simulink model "pid_simulink"  (R2014b)
settings: Solver=ode45  StartTime=0.0  StopTime=10  RelTol=1e-3
values from neighbouring files (symbols this model uses):
  Bm = 0.01    [d_1_dc_motor_parameter.m]    (also in d_2_draw_wt_theta_real.m; d_2_draw_wt_theta_tf.m; d_4_dc_motor_bar_parameter.m; plot.m)
  Jm = 0.000052    (= 5.2e-05)    [d_1_dc_motor_parameter.m]    (also in d_2_draw_wt_theta_real.m; d_2_draw_wt_theta_tf.m; d_4_dc_motor_bar_parameter.m; plot.m)
  Ke = 0.235    [d_1_dc_motor_parameter.m]    (also in d_2_draw_wt_theta_real.m; d_2_draw_wt_theta_tf.m; d_4_dc_motor_bar_parameter.m; plot.m)
  Kt = 0.235    [d_1_dc_motor_parameter.m]    (also in d_2_draw_wt_theta_real.m; d_2_draw_wt_theta_tf.m; d_4_dc_motor_bar_parameter.m; plot.m)
  La = 0.23    [d_1_dc_motor_parameter.m]    (also in d_2_draw_wt_theta_real.m; d_2_draw_wt_theta_tf.m; d_4_dc_motor_bar_parameter.m; plot.m)
  Ra = 2    [d_1_dc_motor_parameter.m]    (also in d_2_draw_wt_theta_real.m; d_2_draw_wt_theta_tf.m; d_4_dc_motor_bar_parameter.m; plot.m)
libraries: simulink x3
settings Model: Creator=Admin  LastModifiedBy=Admin

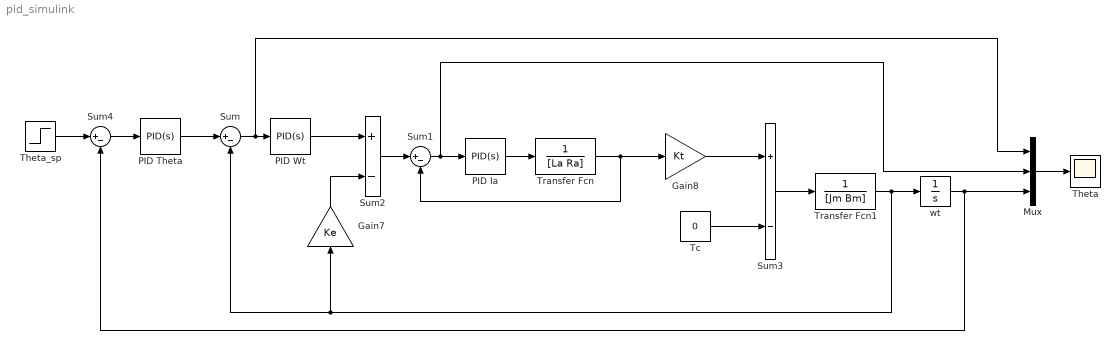
== system pid_simulink ==
  Gain7 : Gain  Gain=Ke
  Gain8 : Gain  Gain=Kt
  Mux : Mux  Inputs=3
  PID Ia : simulink/Continuous/PID Controller  Controller=PID  TimeDomain=Continuous-time  SampleTime=-1  IntegratorMethod=Forward Euler  FilterMethod=Forward Euler  Form=Parallel  P=0.2  I=0.4  D=0  N=0  InitialConditionSource=internal  InitialConditionForIntegrator=0  InitialConditionForFilter=0  ExternalReset=none  LimitOutput=off  UpperSaturationLimit=inf  LowerSaturationLimit=-inf  LinearizeAsGain=on  AntiWindupMode=none  Kb=1  TrackingMode=off  Kt=1  PParamMin=[]  PParamMax=[]  IParamMin=[]  IParamMax=[]  DParamMin=[]  DParamMax=[]  NParamMin=[]  NParamMax=[]  KbParamMin=[]  KbParamMax=[]  KtParamMin=[]  KtParamMax=[]  POutMin=[]  POutMax=[]  IOutMin=[]  IOutMax=[]  DOutMin=[]  DOutMax=[]  NOutMin=[]  NOutMax=[]  KbOutMin=[]  KbOutMax=[]  KtOutMin=[]  KtOutMax=[]  IntegratorOutMin=[]  IntegratorOutMax=[]  FilterOutMin=[]  FilterOutMax=[]  SumOutMin=[]  SumOutMax=[]  SumI1OutMin=[]  SumI1OutMax=[]  SumI2OutMin=[]  SumI2OutMax=[]  SumI3OutMin=[]  SumI3OutMax=[]  SumDOutMin=[]  SumDOutMax=[]  SaturationOutMin=[]  SaturationOutMax=[]  IntegratorContinuousStateAttributes=''  IntegratorStateMustResolveToSignalObject=off  IntegratorRTWStateStorageClass=Auto  FilterContinuousStateAttributes=''  FilterStateMustResolveToSignalObject=off  FilterRTWStateStorageClass=Auto  DifferentiatorICPrevScaledInput=0  DifferentiatorOutMin=[]  DifferentiatorOutMax=[]  UseFilter=on
  PID Theta : simulink/Continuous/PID Controller  Controller=PID  TimeDomain=Continuous-time  SampleTime=-1  IntegratorMethod=Forward Euler  FilterMethod=Forward Euler  Form=Parallel  P=10  I=0  D=0  N=0  InitialConditionSource=internal  InitialConditionForIntegrator=0  InitialConditionForFilter=0  ExternalReset=none  LimitOutput=off  UpperSaturationLimit=inf  LowerSaturationLimit=-inf  LinearizeAsGain=on  AntiWindupMode=none  Kb=1  TrackingMode=off  Kt=1  PParamMin=[]  PParamMax=[]  IParamMin=[]  IParamMax=[]  DParamMin=[]  DParamMax=[]  NParamMin=[]  NParamMax=[]  KbParamMin=[]  KbParamMax=[]  KtParamMin=[]  KtParamMax=[]  POutMin=[]  POutMax=[]  IOutMin=[]  IOutMax=[]  DOutMin=[]  DOutMax=[]  NOutMin=[]  NOutMax=[]  KbOutMin=[]  KbOutMax=[]  KtOutMin=[]  KtOutMax=[]  IntegratorOutMin=[]  IntegratorOutMax=[]  FilterOutMin=[]  FilterOutMax=[]  SumOutMin=[]  SumOutMax=[]  SumI1OutMin=[]  SumI1OutMax=[]  SumI2OutMin=[]  SumI2OutMax=[]  SumI3OutMin=[]  SumI3OutMax=[]  SumDOutMin=[]  SumDOutMax=[]  SaturationOutMin=[]  SaturationOutMax=[]  IntegratorContinuousStateAttributes=''  IntegratorStateMustResolveToSignalObject=off  IntegratorRTWStateStorageClass=Auto  FilterContinuousStateAttributes=''  FilterStateMustResolveToSignalObject=off  FilterRTWStateStorageClass=Auto  DifferentiatorICPrevScaledInput=0  DifferentiatorOutMin=[]  DifferentiatorOutMax=[]  UseFilter=on
  PID Wt : simulink/Continuous/PID Controller  Controller=PID  TimeDomain=Continuous-time  SampleTime=-1  IntegratorMethod=Forward Euler  FilterMethod=Forward Euler  Form=Parallel  P=1  I=2  D=0  N=0  InitialConditionSource=internal  InitialConditionForIntegrator=0  InitialConditionForFilter=0  ExternalReset=none  LimitOutput=off  UpperSaturationLimit=inf  LowerSaturationLimit=-inf  LinearizeAsGain=on  AntiWindupMode=none  Kb=1  TrackingMode=off  Kt=1  PParamMin=[]  PParamMax=[]  IParamMin=[]  IParamMax=[]  DParamMin=[]  DParamMax=[]  NParamMin=[]  NParamMax=[]  KbParamMin=[]  KbParamMax=[]  KtParamMin=[]  KtParamMax=[]  POutMin=[]  POutMax=[]  IOutMin=[]  IOutMax=[]  DOutMin=[]  DOutMax=[]  NOutMin=[]  NOutMax=[]  KbOutMin=[]  KbOutMax=[]  KtOutMin=[]  KtOutMax=[]  IntegratorOutMin=[]  IntegratorOutMax=[]  FilterOutMin=[]  FilterOutMax=[]  SumOutMin=[]  SumOutMax=[]  SumI1OutMin=[]  SumI1OutMax=[]  SumI2OutMin=[]  SumI2OutMax=[]  SumI3OutMin=[]  SumI3OutMax=[]  SumDOutMin=[]  SumDOutMax=[]  SaturationOutMin=[]  SaturationOutMax=[]  IntegratorContinuousStateAttributes=''  IntegratorStateMustResolveToSignalObject=off  IntegratorRTWStateStorageClass=Auto  FilterContinuousStateAttributes=''  FilterStateMustResolveToSignalObject=off  FilterRTWStateStorageClass=Auto  DifferentiatorICPrevScaledInput=0  DifferentiatorOutMin=[]  DifferentiatorOutMax=[]  UseFilter=on
  Sum : Sum  Inputs=|+-
  Sum1 : Sum  Inputs=|+-
  Sum2 : Sum  Inputs=+-
  Sum3 : Sum  Inputs=+-
  Sum4 : Sum  Inputs=|+-
  Tc : Constant  Value=0
  Theta : Scope
      settings: TimeRange=1  YMin=-1  YMax=1  SaveName=ScopeData4
  Theta_sp : Step  Time=0  After=100  SampleTime=0
  Transfer Fcn : TransferFcn  Denominator=[La Ra]
  Transfer Fcn1 : TransferFcn  Denominator=[Jm Bm]
  wt : Integrator
  wires:
  Sum/1 -> Mux/1, PID Wt/1
  Gain7/1 -> Sum2/2
  Gain8/1 -> Sum3/1
  Transfer Fcn/1 -> Sum1/2, Gain8/1
  PID Wt/1 -> Sum2/1
  Sum3/1 -> Transfer Fcn1/1
  Transfer Fcn1/1 -> Gain7/1, Sum/2, wt/1
  wt/1 -> Mux/3, Sum4/2
  Sum1/1 -> Mux/2, PID Ia/1
  Sum2/1 -> Sum1/1
  PID Ia/1 -> Transfer Fcn/1
  Sum4/1 -> PID Theta/1
  Theta_sp/1 -> Sum4/1
  PID Theta/1 -> Sum/1
  Tc/1 -> Sum3/2
  Mux/1 -> Theta/1
